simulink model "reactivePTO"  (R2022b)
settings: Solver=ode45  StartTime=0  StopTime=100  FixedStep=0.01  MaxStep=0.01  RelTol=1e-3  EnableMultiTasking=on
values from neighbouring files (symbols this model uses):
  gearRatio = 100    [wecSimInputFile.m]
  generatorJ = 20    [wecSimInputFile.m]
  generatorR = .483    (= 0.483)    [wecSimInputFile.m]
  Kt = 7.186    [wecSimInputFile.m]
  shaftMechDamping = 1    [wecSimInputFile.m]
  simu = simulationClass()    [wecSimInputFile.m]
  tcControl = generatorL/generatorR    (= 0.0108136645963)    [wecSimInputFile.m]
undefined symbols (not defined in the file or in its folder): body, controller, geometry, hydroData, magnitude, pto
libraries: WECSim_Lib_Body_Elements x1, WECSim_Lib_Frames x1, WECSim_Lib_PTOs x1
settings Model: Creator=mlawson  LastModifiedBy=jtgrasb
settings SolverCC: ZeroCrossControl=DisableAll  AlgebraicLoopSolver=LineSearch  AutoInsertRateTranBlk=on
settings DataIOCC: SaveFormat=Array  SaveOutput=off  SaveTime=off  ReturnWorkspaceOutputs=off
settings OptimizationCC: LifeSpan=inf  SimCompilerOptimization=on
settings DebuggingCC: UnderspecifiedInitializationDetection=Classic  MergeDetectMultiDrivingBlocksExec=none  SolverPrmCheckMsg=warning  UnconnectedInputMsg=warning  UnconnectedOutputMsg=warning  UnconnectedLineMsg=warning  AllowSymbolicDim=off  StateNameClashWarn=warning  SFUnexpectedBacktrackingDiag=warning  SFNoUnconditionalDefaultTransitionDiag=warning  SFExecutionAtInitializationDiag=none  SFMachineParentedDataDiag=warning  ArithmeticOperatorsInVariantConditions=warning
settings HardwareCC: ProdBitPerPointer=32  ProdBitPerSizeT=32  ProdBitPerPtrDiffT=32  ProdLargestAtomicFloat=None  ProdIntDivRoundTo=Undefined  ProdEndianess=Unspecified  ProdWordSize=32  ProdHWDeviceType=32-bit Generic
settings ModelReferenceCC: EnableRefExpFcnMdlSchedulingChecks=on  PropagateSignalLabelsOutOfModel=off
settings SFSimCC: SimUseLocalCustomCode=off  CustomCodeUndefinedFunction=UseInterfaceOnly
settings RTWCC: RTWUseLocalCustomCode=off  DLArmComputeVersion=19.05
settings CodeAppCC: StateflowObjectComments=on
settings GRTTargetCC: TargetLangStandard=C89/C90 (ANSI)
settings ConfigComp: CovMetricSettings=dw  CovSaveCumulativeToWorkspaceVar=on  CovSaveSingleToWorkspaceVar=on  CovExternalEMLEnable=off  CovSFcnEnable=off
settings SimscapeCC: SimscapeNormalizeSystem=off
settings ConfigurationSet: Description=SimMechanics 2G
settings ExplorerConfigSet: SimMechanicsOpenEditorOnUpdate=off  InternalSimMechanicsExplorerSettings="<ExplorerConfiguration><canonicalview>default</canonicalview><TilePanel><TileInfo><Tiles Columns=\"1\" Count=\"1\" Rows=\"1\"><Column Left=\"2\" Weight=\"1\"/><Column Left=\"1335\"/><Row Top=\"2\" Weight=\"1\"/><Row Top=\"911\"/><Tile Height=\"1\" Width=\"1\" X=\"0\" Y=\"0\"/></Tiles></TileInfo><SceneInfo><SceneViewer><BGColor><R>0.60000002384185791</R><G>0.60000002384185791</G><B>0.60000002384185791</B></BGColor><Camera><Position><X>365.37645888990272</X><Y>-369.82486814446582</Y><Z>359.64809521743916</Z></Position><Center><X>-6.7351450971904585</X><Y>2.2867358426280204</Y><Z>-12.463508769654169</Z></Center><Up><X>-0.40824829046386307</X><Y>0.40824829046386307</Y><Z>0.81649658092772615</Z></Up><Left>-57.820127362122818</Left><Right>57.820127362122818</Right><Bottom>-38.308817187253304</Bottom><Top>38.308817187253304</Top></Camera></SceneViewer></SceneInfo></TilePanel></ExplorerConfiguration>"

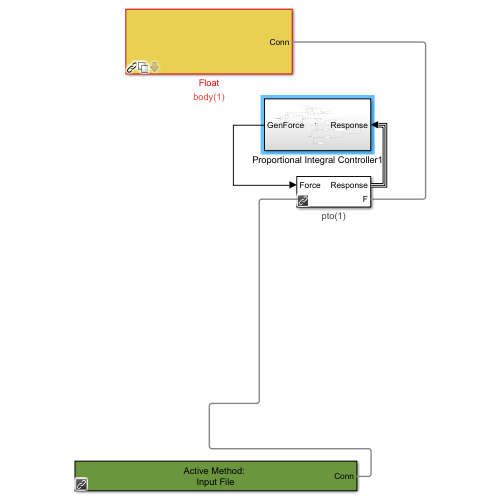
[thumbnail: Simulink's stored preview of the top-level diagram]
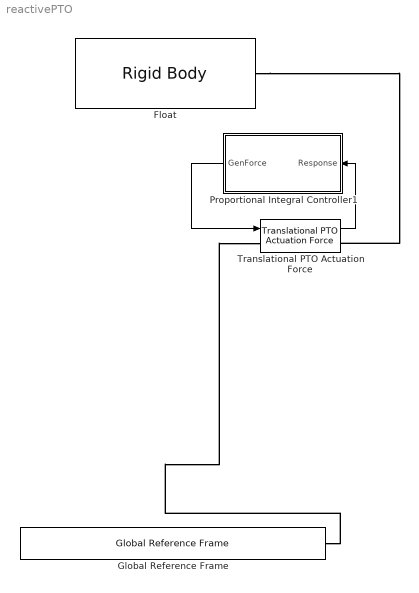
== system reactivePTO ==
  Float : WECSim_Lib_Body_Elements/Rigid Body  body=body(1)  h5File=hydroData/*.h5  geometryFile=geometry/*.stl  mass=0  inertia=0 0 0  inertiaProducts=0 0 0  nonHydro=0  nonlinearHydro=0  centerGravity=0 0 0  centerBuoyancy=0 0 0  dof=6  volume=0  displacement=0 0 0  axis=0 1 0  angle=0  option=0  cd=0 0 0  ca=0 0 0  area=0 0 0  VME=0  rgME=0 0 0  z=0 0 1
  Global Reference Frame : WECSim_Lib_Frames/Global Reference Frame  waves=waves  simu=simu  InputMethod=Input File  InputFile=wecSimInputFile.m  mode=normal  explorer=off  solver=ode4  startTime=0  rampTime=100  endTime=400  dt=0.1  cicEndTime=60  stateSpace=0  WaveClass=regular  height=2.5  period=8  elevationFile=NOT DEFINED  spectrumFile=NOT DEFINED  direction=0  spread=1  spectrumType=NOT DEFINED  phaseSeed=0  option=EqualEnergy
  Proportional Integral Controller1 : Subsystem
  Translational PTO Actuation Force : WECSim_Lib_PTOs/Translational PTO Actuation Force  pto=pto(1)  loc="0  0  0"  stiffness=0  damping=0  equilibriumPosition=0  pretension=0  displacement=0 0 0  y=0 1 0  z=0 0 1  upperLimitSpecify=off  upperLimitBound=0  upperLimitTransitionRegionWidth=0  upperLimitStiffness=0  upperLimitDamping=0  lowerLimitSpecify=off  lowerLimitBound=0  lowerLimitTransitionRegionWidth=0  lowerLimitStiffness=0  lowerLimitDamping=0
      settings: AttributesFormatString=%<pto>
  wires:
  Proportional Integral Controller1/1(GenForce) -> Translational PTO Actuation Force/1
  Translational PTO Actuation Force/1 -> Proportional Integral Controller1/1(Response)
  connections:
  Global Reference Frame/RConn1 -- Translational PTO Actuation Force/LConn1
  Float/RConn1 -- Translational PTO Actuation Force/RConn1

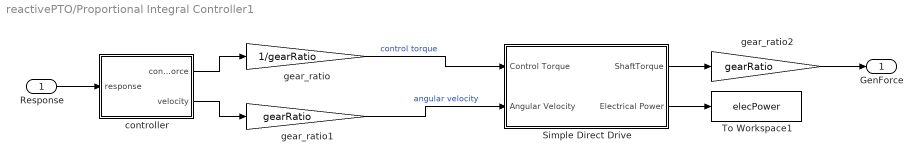
== system reactivePTO/Proportional Integral Controller1 ==
  Response : Inport
  Simple Direct Drive : Subsystem  TreatAsAtomicUnit=on
  To Workspace1 : ToWorkspace  VariableName=elecPower  SaveFormat=Timeseries  SampleTime=-1
  controller : Subsystem
  gear_ratio : Gain  Gain=1/gearRatio
  gear_ratio1 : Gain  Gain=gearRatio
  gear_ratio2 : Gain  Gain=gearRatio
  GenForce : Outport
  wires:
  gear_ratio1/1 -> Simple Direct Drive/2(Angular Velocity)  "angular velocity"
  Simple Direct Drive/1(ShaftTorque) -> gear_ratio2/1
  Simple Direct Drive/2(Electrical Power) -> To Workspace1/1
  gear_ratio2/1 -> GenForce/1
  gear_ratio/1 -> Simple Direct Drive/1(Control Torque)  "control torque"
  Response/1 -> controller/1(response)
  controller/1(controlForce) -> gear_ratio/1
  controller/2(velocity) -> gear_ratio1/1

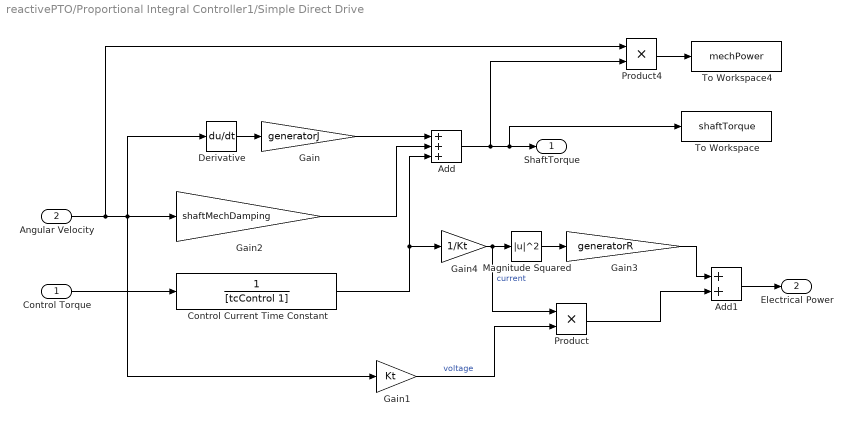
== system reactivePTO/Proportional Integral Controller1/Simple Direct Drive ==
  Control Torque : Inport
  Angular Velocity : Inport  Port=2
  Add : Sum  Inputs=+++
  Add1 : Sum
  Control Current Time Constant : TransferFcn  Denominator=[tcControl 1]
  Derivative : Derivative  CoefficientInTFapproximation=1000*2*pi
  Gain : Gain  Gain=generatorJ
  Gain1 : Gain  Gain=Kt
  Gain2 : Gain  Gain=shaftMechDamping
  Gain3 : Gain  Gain=generatorR
  Gain4 : Gain  Gain=1/Kt
  Magnitude Squared : Math  Operator=magnitude^2
  Product : Product
  Product4 : Product
  To Workspace : ToWorkspace  VariableName=shaftTorque  SaveFormat=Timeseries  SampleTime=-1
  To Workspace4 : ToWorkspace  VariableName=mechPower  SaveFormat=Timeseries  SampleTime=-1
  ShaftTorque : Outport
  Electrical Power : Outport  Port=2
  wires:
  Derivative/1 -> Gain/1
  Control Torque/1 -> Control Current Time Constant/1
  Gain/1 -> Add/1
  Control Current Time Constant/1 -> Add/3, Gain4/1
  Gain2/1 -> Add/2
  Add/1 -> Product4/2, To Workspace/1, ShaftTorque/1
  Angular Velocity/1 -> Product4/1, Gain1/1, Gain2/1, Derivative/1
  Magnitude Squared/1 -> Gain3/1
  Add1/1 -> Electrical Power/1
  Product/1 -> Add1/2
  Gain3/1 -> Add1/1
  Gain4/1 -> Product/1, Magnitude Squared/1  "current"
  Gain1/1 -> Product/2  "voltage"
  Product4/1 -> To Workspace4/1

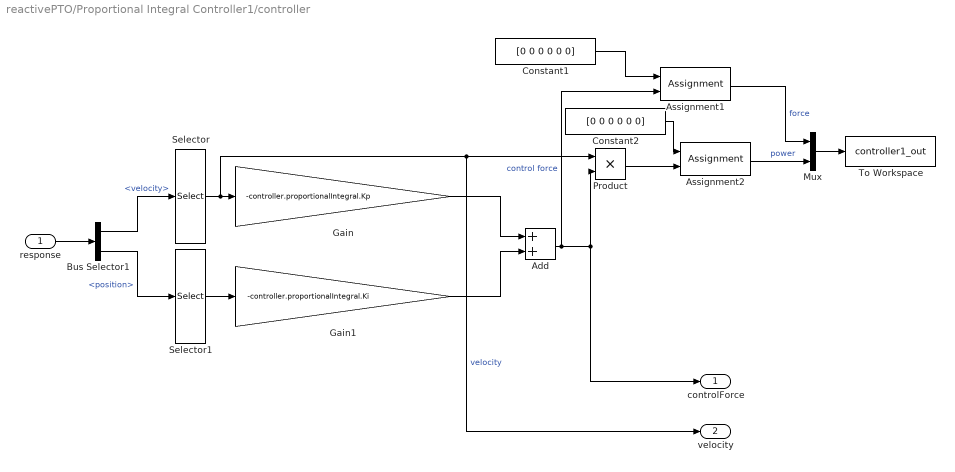
== system reactivePTO/Proportional Integral Controller1/controller ==
  response : Inport
  Add : Sum
  Assignment1 : Assignment  IndexOptions=Index vector (dialog)  Indices=3  OutputSizes=1
  Assignment2 : Assignment  IndexOptions=Index vector (dialog)  Indices=3  OutputSizes=1
  Bus Selector1 : BusSelector  OutputSignals=velocity,position
  Constant1 : Constant  Value=[0 0 0 0 0 0]
  Constant2 : Constant  Value=[0 0 0 0 0 0]
  Gain : Gain  Gain=-controller.proportionalIntegral.Kp
  Gain1 : Gain  Gain=-controller.proportionalIntegral.Ki
  Mux : Mux  Inputs=2
  Product : Product
  Selector : Selector  InputPortWidth=6  IndexOptions=Index vector (dialog)  Indices=3  OutputSizes=1
  Selector1 : Selector  InputPortWidth=6  IndexOptions=Index vector (dialog)  Indices=3  OutputSizes=1
  To Workspace : ToWorkspace  VariableName=controller1_out  SaveFormat=Structure With Time  SampleTime=simu.dtOut
  controlForce : Outport
  velocity : Outport  Port=2
  wires:
  response/1 -> Bus Selector1/1
  Gain1/1 -> Add/2
  Constant1/1 -> Assignment1/1
  Constant2/1 -> Assignment2/1
  Assignment2/1 -> Mux/2  "power"
  Bus Selector1/1 -> Selector/1  "<velocity>"
  Bus Selector1/2 -> Selector1/1  "<position>"
  Add/1 -> Assignment1/2, controlForce/1, Product/2  "control force"
  Assignment1/1 -> Mux/1  "force"
  Selector1/1 -> Gain1/1
  Selector/1 -> velocity/1, Product/1, Gain/1  "velocity"
  Product/1 -> Assignment2/2
  Mux/1 -> To Workspace/1
  Gain/1 -> Add/1
